simulink model "H036_Buck_Boost_Converter_DC_motor"  (R2021a)
settings: Solver=VariableStepAuto  StartTime=0.0  StopTime=10  RelTol=1e-3
libraries: simulink x2
settings Model: Creator=Pallavi  LastModifiedBy=Pallavi

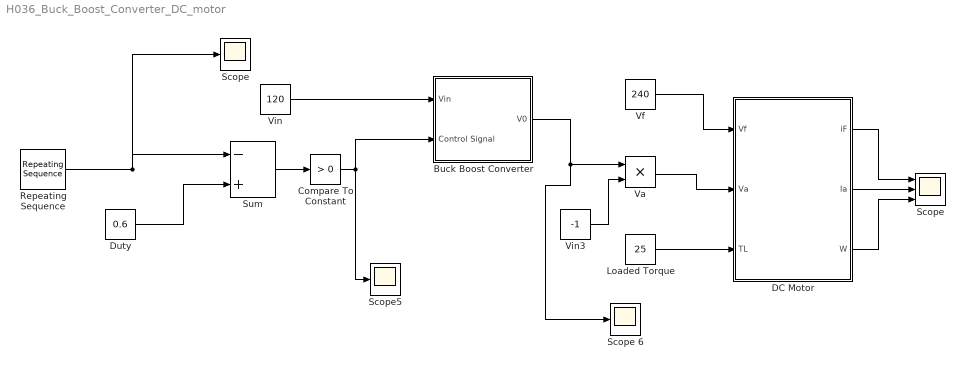
== system H036_Buck_Boost_Converter_DC_motor ==
  Buck Boost Converter : Subsystem
  Compare To Constant : simulink/Logic and Bit Operations/Compare To Constant  relop=>  const=0  OutDataTypeStr=boolean
  DC Motor : Subsystem
  Duty : Constant  Value=0.6
  Loaded Torque : Constant  Value=25
  "Repeating Sequence " : simulink/Sources/Repeating Sequence  rep_seq_t=[0 2]  rep_seq_y=[0 2]
  Scope : Scope
  "Scope " : Scope  NumInputPorts=3
  Scope 6 : Scope
  "Scope5 " : Scope
  Sum : Sum  Inputs=|-+
  Va : Product
  Vf : Constant  Value=240
  Vin : Constant  Value=120
  Vin3 : Constant  Value=-1
  wires:
  "Repeating Sequence "/1 -> Scope/1, Sum/1
  Duty/1 -> Sum/2
  Sum/1 -> Compare To Constant/1
  Compare To Constant/1 -> "Scope5 "/1, Buck Boost Converter/2(Control Signal)
  Vin/1 -> Buck Boost Converter/1(Vin)
  Buck Boost Converter/1(V0) -> Scope 6/1, Va/1
  Vin3/1 -> Va/2
  Vf/1 -> DC Motor/1(Vf)
  Va/1 -> DC Motor/2(Va)
  Loaded Torque/1 -> DC Motor/3(TL)
  DC Motor/1(iF) -> "Scope "/1
  DC Motor/2(Ia) -> "Scope "/2
  DC Motor/3(W) -> "Scope "/3

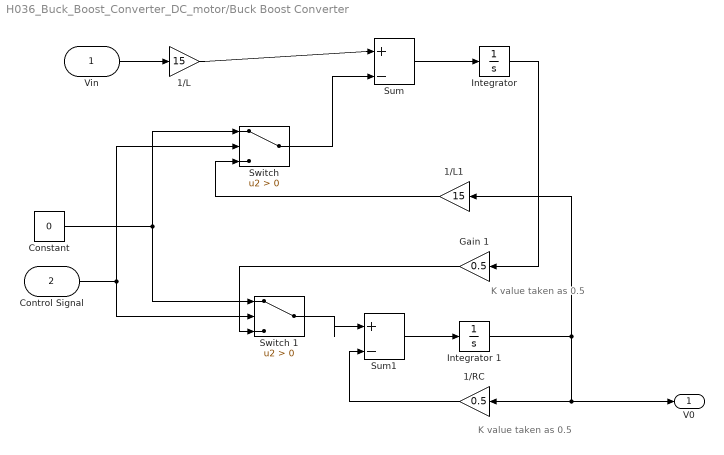
== system H036_Buck_Boost_Converter_DC_motor/Buck Boost Converter ==
  note: K value taken as 0.5
  note: K value taken as 0.5
  Vin : Inport
  Control Signal : Inport  Port=2
  1/L : Gain  Gain=15
  1/L1 : Gain  Gain=15
  1/RC : Gain  Gain=0.5
  "Constant " : Constant  Value=0
  Gain 1 : Gain  Gain=0.5
  "Integrator " : Integrator
  Integrator 1 : Integrator
  Sum : Sum  Inputs=|+-
  Sum1 : Sum  Inputs=|+-
  "Switch " : Switch  Criteria=u2 > Threshold
  Switch 1 : Switch  Criteria=u2 > Threshold
  V0 : Outport
  wires:
  Integrator 1/1 -> 1/RC/1, V0/1, 1/L1/1
  Sum/1 -> "Integrator "/1
  1/RC/1 -> Sum1/2
  Switch 1/1 -> Sum1/1
  "Switch "/1 -> Sum/2
  "Integrator "/1 -> Gain 1/1
  Sum1/1 -> Integrator 1/1
  Gain 1/1 -> Switch 1/3
  1/L1/1 -> "Switch "/3
  "Constant "/1 -> Switch 1/1, "Switch "/1
  Control Signal/1 -> Switch 1/2, "Switch "/2
  Vin/1 -> 1/L/1
  1/L/1 -> Sum/1

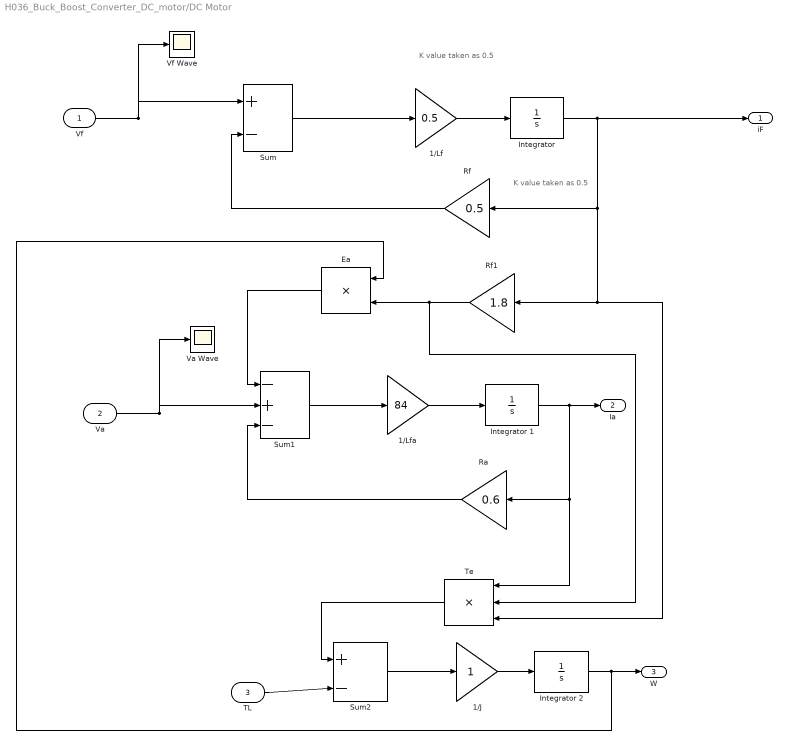
== system H036_Buck_Boost_Converter_DC_motor/DC Motor ==
  note: K value taken as 0.5
  note: K value taken as 0.5
  Vf : Inport
  Va : Inport  Port=2
  TL : Inport  Port=3
  1/J : Gain
  1/Lf : Gain  Gain=0.5
  1/Lfa : Gain  Gain=84
  Ea : Product
  "Integrator " : Integrator
  Integrator 1 : Integrator
  Integrator 2 : Integrator
  Ra : Gain  Gain=0.6
  Rf : Gain  Gain=0.5
  Rf1 : Gain  Gain=1.8
  Sum : Sum  Inputs=|+-
  Sum1 : Sum  Inputs=|-+-
  Sum2 : Sum  Inputs=|+-
  Te : Product  Inputs=3
  Va Wave : Scope
  Vf Wave : Scope
  iF : Outport
  Ia : Outport  Port=2
  W : Outport  Port=3
  wires:
  Sum2/1 -> 1/J/1
  Va/1 -> Sum1/2, Va Wave/1
  TL/1 -> Sum2/2
  Integrator 2/1 -> Ea/1, W/1
  Te/1 -> Sum2/1
  1/Lfa/1 -> Integrator 1/1
  Ea/1 -> Sum1/1
  Ra/1 -> Sum1/3
  "Integrator "/1 -> Rf1/1, Te/3, Rf/1, iF/1
  1/J/1 -> Integrator 2/1
  Rf1/1 -> Te/2, Ea/2
  Sum1/1 -> 1/Lfa/1
  1/Lf/1 -> "Integrator "/1
  Rf/1 -> Sum/2
  Integrator 1/1 -> Te/1, Ra/1, Ia/1
  Vf/1 -> Vf Wave/1, Sum/1
  Sum/1 -> 1/Lf/1
